simulink model "comparison_CT_DT"  (R2020b)
settings: Solver=ode45  StartTime=0.0  StopTime=10.0  MaxStep=0.5e-3  RelTol=1e-6
values from neighbouring files (symbols this model uses):
  s0 = C0_features(:)    [init.m]
  s_star = C_features_desired(:)    [init.m]
  Ts = 0.1    [init.m]
settings Model: Creator=marco  LastModifiedBy=marco

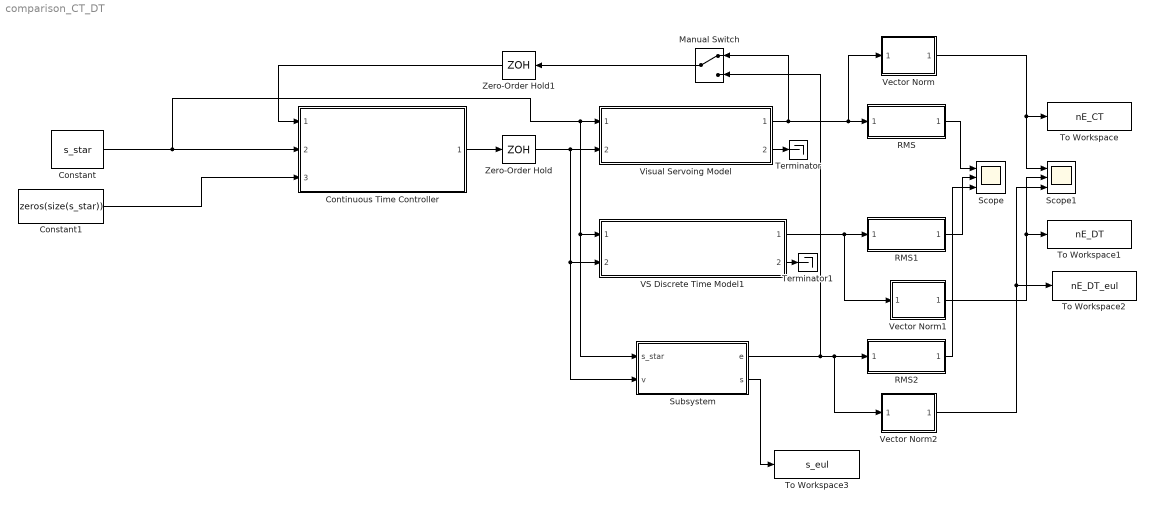
== system comparison_CT_DT ==
  Constant : Constant  Value=s_star
  Constant1 : Constant  Value=zeros(size(s_star))
  Continuous Time Controller : Subsystem  ReferencedSubsystem=continuous_time_controller  lambda=lambda  forward_action_enabled=off
  Manual Switch : ManualSwitch
  RMS : Subsystem  ReferencedSubsystem=RMS
  RMS1 : Subsystem  ReferencedSubsystem=RMS
  RMS2 : Subsystem  ReferencedSubsystem=RMS
  Scope : Scope  NumInputPorts=3
  Scope1 : Scope  NumInputPorts=3
  Subsystem : Subsystem  mask{s0=s0, Ts=Ts, noise_perc=0}
      mask Display:
      | disp('s_{k+1}=s_{k}+T L(s_k)v_k','texmode', 'on')
      | port_label('output',1,'e','texmode', 'on')
      | port_label('output',2,'s','texmode', 'on')
      | port_label('input',1,'s^*','texmode', 'on')
      | port_label('input',2,'v','texmode', 'on')
  Terminator : Terminator
  Terminator1 : Terminator
  To Workspace : ToWorkspace  VariableName=nE_CT  SaveFormat=Timeseries  SampleTime=-1
  To Workspace1 : ToWorkspace  VariableName=nE_DT  SaveFormat=Timeseries  SampleTime=-1
  To Workspace2 : ToWorkspace  VariableName=nE_DT_eul  SaveFormat=Timeseries  SampleTime=-1
  To Workspace3 : ToWorkspace  VariableName=s_eul  SaveFormat=Timeseries  SampleTime=-1
  VS Discrete Time Model1 : Subsystem  ReferencedSubsystem=VS_DiscreteTimeModel  s0=s0  Ts=Ts  noise_perc=0
  Vector Norm : Subsystem  ReferencedSubsystem=Norm
  Vector Norm1 : Subsystem  ReferencedSubsystem=Norm
  Vector Norm2 : Subsystem  ReferencedSubsystem=Norm
  Visual Servoing Model : Subsystem  ReferencedSubsystem=Features_System  s0=s0  noise_perc=0  noise_sample_time=1
  Zero-Order Hold : ZeroOrderHold  SampleTime=Ts
  Zero-Order Hold1 : ZeroOrderHold  SampleTime=Ts
  wires:
  Visual Servoing Model/1 -> Manual Switch/1, Vector Norm/1, RMS/1
  RMS/1 -> Scope/1
  Continuous Time Controller/1 -> Zero-Order Hold/1
  Constant/1 -> Subsystem/1(s_star), VS Discrete Time Model1/1, Visual Servoing Model/1, Continuous Time Controller/2
  Constant1/1 -> Continuous Time Controller/3
  Zero-Order Hold1/1 -> Continuous Time Controller/1
  VS Discrete Time Model1/1 -> Vector Norm1/1, RMS1/1
  RMS1/1 -> Scope/2
  Zero-Order Hold/1 -> Subsystem/2(v), VS Discrete Time Model1/2, Visual Servoing Model/2
  Manual Switch/1 -> Zero-Order Hold1/1
  Vector Norm/1 -> To Workspace/1, Scope1/1
  Vector Norm1/1 -> To Workspace1/1, Scope1/2
  RMS2/1 -> Scope/3
  Vector Norm2/1 -> To Workspace2/1, Scope1/3
  Subsystem/1(e) -> Manual Switch/2, Vector Norm2/1, RMS2/1
  Subsystem/2(s) -> To Workspace3/1
  Visual Servoing Model/2 -> Terminator/1
  VS Discrete Time Model1/2 -> Terminator1/1

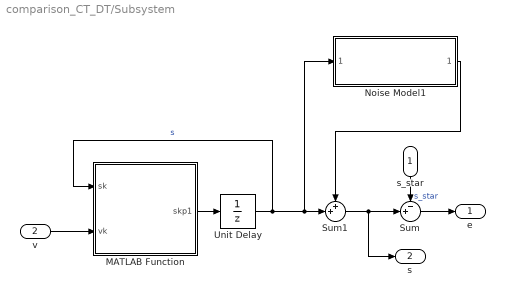
== system comparison_CT_DT/Subsystem ==
  s_star : Inport
  v : Inport  Port=2
  MATLAB Function : MATLAB Function  TreatAsAtomicUnit=on
  Noise Model1 : Subsystem  ReferencedSubsystem=VSNoiseModel  noise_perc=noise_perc  noise_sample_time=Ts
  Sum : Sum  Inputs=-+|
  Sum1 : Sum  Inputs=++|
  Unit Delay : UnitDelay  InitialCondition=s0  SampleTime=Ts  HasFrameUpgradeWarning=on
  e : Outport
  s : Outport  Port=2
  wires:
  v/1 -> MATLAB Function/2(vk)
  Noise Model1/1 -> Sum1/1
  Sum/1 -> e/1
  s_star/1 -> Sum/1  "s_star"
  Sum1/1 -> Sum/2, s/1
  MATLAB Function/1(skp1) -> Unit Delay/1
  Unit Delay/1 -> MATLAB Function/1(sk), Noise Model1/1, Sum1/2  "s"

== matlab function comparison_CT_DT/Subsystem/MATLAB Function ==
  data: sk input; skp1 output; vk input; Ts parameter
function skp1 = fcn(sk, vk,Ts)

sdot = computeL(sk)*vk;
skp1 = sk + Ts*sdot;
